simulink model "L1E4pt2_DC_Motor_Speed_Model"  (R2019b)
settings: Solver=VariableStepAuto  StartTime=0.0  StopTime=10.0  RelTol=1e-3
libraries: fl_lib x10, nesl_utility x5
settings Model: Creator=Callum  LastModifiedBy=Callum

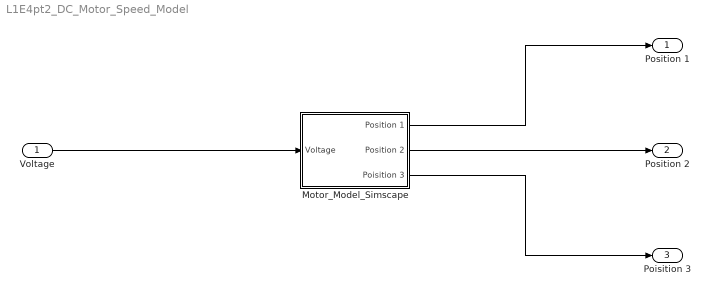
== system L1E4pt2_DC_Motor_Speed_Model ==
  Voltage : Inport
  Motor_Model_Simscape : Subsystem
  Position 1 : Outport
  Position 2 : Outport  Port=2
  Poisition 3 : Outport  Port=3
  wires:
  Voltage/1 -> Motor_Model_Simscape/1(Voltage)
  Motor_Model_Simscape/1(Position 1) -> Position 1/1
  Motor_Model_Simscape/2(Position 2) -> Position 2/1
  Motor_Model_Simscape/3(Poisition 3) -> Poisition 3/1

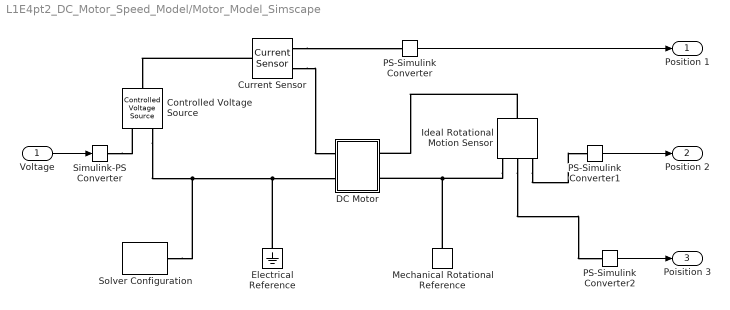
== system L1E4pt2_DC_Motor_Speed_Model/Motor_Model_Simscape ==
  Voltage : Inport
  "Controlled Voltage Source " : fl_lib/Electrical/Electrical Sources/Controlled Voltage Source
  "Current Sensor " : fl_lib/Electrical/Electrical Sensors/Current Sensor
  DC Motor : Subsystem
  "Electrical Reference " : fl_lib/Electrical/Electrical Elements/Electrical Reference
  "Ideal Rotational Motion Sensor " : fl_lib/Mechanical/Mechanical Sensors/Ideal Rotational Motion Sensor  offset=0 rad
  "Mechanical Rotational Reference " : fl_lib/Mechanical/Rotational Elements/Mechanical Rotational Reference
  PS-Simulink Converter : nesl_utility/PS-Simulink Converter  PhysicalDomain=network_engine_domain  SubClassName=ps_output  LeftPortType=input  RightPortType=output  PseudoPeriodic=off  Frequencies=[]  Unit=inherit  AffineConversion=off
  PS-Simulink Converter1 : nesl_utility/PS-Simulink Converter  PhysicalDomain=network_engine_domain  SubClassName=ps_output  LeftPortType=input  RightPortType=output  PseudoPeriodic=off  Frequencies=[]  Unit=inherit  AffineConversion=off
  PS-Simulink Converter2 : nesl_utility/PS-Simulink Converter  PhysicalDomain=network_engine_domain  SubClassName=ps_output  LeftPortType=input  RightPortType=output  PseudoPeriodic=off  Frequencies=[]  Unit=inherit  AffineConversion=off
  "Simulink-PS Converter " : nesl_utility/Simulink-PS Converter  PhysicalDomain=network_engine_domain  SubClassName=ps_input  LeftPortType=input  RightPortType=output  PseudoPeriodic=off  Frequencies=[]  NoiseDistribution=none  NoiseParameters=[]  Unit=1  AffineConversion=off  FilteringAndDerivatives=provide  SimscapeFilterOrder=1  InputFilterTimeConstant=0.001  UdotUserProvided=0
  "Solver Configuration " : nesl_utility/Solver Configuration  PhysicalDomain=network_engine_domain  SubClassName=solver  LeftPortType=input  RightPortType=generic  Tones=[]  Harmonics=[]  SimulateNoise=off  Profile=off  UseLocalSampling=off  EnableSwitchedLinearOptims=on  FrequencyDomain=off  UseCCode=off  RelTol=0.001  AbsTol=1e-06  MinStep=1e-09  ToWorkspace=off  RevertToSquareIcSolve=off  NumHomotopyIterations=100  PhasorMode=off  PhasorModeNumHarmonics=1  DoDC=off  ResidualTolerance=1e-09  UseLocalSolver=off  LocalSolverChoice=NE_BACKWARD_EULER_ADVANCER  LocalSolverSampleTime=0.001  DoFixedCost=off  MaxNonlinIter=3  MaxModeIter=2  LinearAlgebra=auto  EquationFormulation=NE_TIME_EF  DelaysMemoryBudget=1024  AutomaticFiltering=on  FilteringTimeConstant=0.001  PartitionStorageMethod=AS_NEEDED  PartitionMemoryBudget=1024  PartitionMethod=ROBUST
  Position 1 : Outport
  Position 2 : Outport  Port=2
  Poisition 3 : Outport  Port=3
  wires:
  Voltage/1 -> "Simulink-PS Converter "/1
  PS-Simulink Converter/1 -> Position 1/1
  PS-Simulink Converter2/1 -> Poisition 3/1
  PS-Simulink Converter1/1 -> Position 2/1
  connections:
  "Current Sensor "/LConn1 -- "Controlled Voltage Source "/LConn1
  "Current Sensor "/RConn2 -- DC Motor/LConn1
  "Current Sensor "/RConn1 -- PS-Simulink Converter/LConn1
  "Controlled Voltage Source "/RConn2 -- "Solver Configuration "/RConn1 -- "Electrical Reference "/LConn1 -- DC Motor/LConn2
  "Ideal Rotational Motion Sensor "/RConn1 -- "Mechanical Rotational Reference "/LConn1 -- DC Motor/RConn2
  "Ideal Rotational Motion Sensor "/RConn2 -- PS-Simulink Converter2/LConn1
  "Ideal Rotational Motion Sensor "/LConn1 -- DC Motor/RConn1
  "Ideal Rotational Motion Sensor "/RConn3 -- PS-Simulink Converter1/LConn1
  "Simulink-PS Converter "/RConn1 -- "Controlled Voltage Source "/RConn1

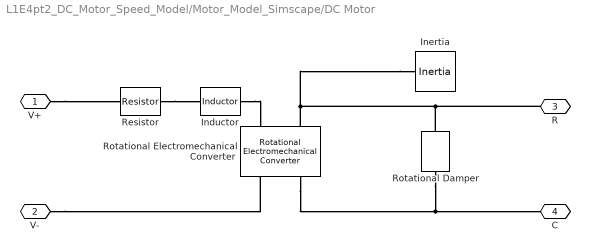
== system L1E4pt2_DC_Motor_Speed_Model/Motor_Model_Simscape/DC Motor ==
  " Inertia" : fl_lib/Mechanical/Rotational Elements/Inertia  inertia=0.01 kg*m^2  w_specify=off  w_priority=High  w=0 rad/s  w_nominal_specify=off  w_nominal_unit=rad/s  w_nominal_value=1  t_specify=off  t_priority=None  t=0 N*m  t_nominal_specify=off  t_nominal_unit=N*m  t_nominal_value=1
  "Inductor " : fl_lib/Electrical/Electrical Elements/Inductor  l=1e-6 H  r=0 Ohm  g=1e-9 1/Ohm  i_specify=off  i_priority=None  i=0 A  i_nominal_specify=off  i_nominal_unit=A  i_nominal_value=1  v_specify=off  v_priority=None  v=0 V  v_nominal_specify=off  v_nominal_unit=V  v_nominal_value=1  i_L_specify=off  i_L_priority=High  i_L=0 A  i_L_nominal_specify=off  i_L_nominal_unit=A  i_L_nominal_value=1
  "Resistor " : fl_lib/Electrical/Electrical Elements/Resistor  R=1 Ohm  i_specify=off  i_priority=None  i=0 A  i_nominal_specify=off  i_nominal_unit=A  i_nominal_value=1  v_specify=off  v_priority=None  v=0 V  v_nominal_specify=off  v_nominal_unit=V  v_nominal_value=1
  "Rotational Electromechanical Converter " : fl_lib/Electrical/Electrical Elements/Rotational Electromechanical Converter  K=0.1 V/(rad/s)  i_specify=off  i_priority=None  i=0 A  i_nominal_specify=off  i_nominal_unit=A  i_nominal_value=1  v_specify=off  v_priority=None  v=0 V  v_nominal_specify=off  v_nominal_unit=V  v_nominal_value=1  t_specify=off  t_priority=None  t=0 N*m  t_nominal_specify=off  t_nominal_unit=N*m  t_nominal_value=1  w_specify=off  w_priority=None  w=0 rad/s  w_nominal_specify=off  w_nominal_unit=rad/s  w_nominal_value=1
      settings: SourceProductName=Simscape
  "Rotational Damper " : fl_lib/Mechanical/Rotational Elements/Rotational Damper  D=0.001 N*m/(rad/s)  w_specify=off  w_priority=None  w=0 rad/s  w_nominal_specify=off  w_nominal_unit=rad/s  w_nominal_value=1  t_specify=off  t_priority=None  t=0 N*m  t_nominal_specify=off  t_nominal_unit=N*m  t_nominal_value=1
  V+ : PMIOPort  Side=Left
  V- : PMIOPort  Port=2  Side=Left
  R : PMIOPort  Port=3  Side=Right
  C : PMIOPort  Port=4  Side=Right
  connections:
  "Inductor "/RConn1 -- "Rotational Electromechanical Converter "/LConn1
  V+/RConn1 -- "Resistor "/LConn1
  " Inertia"/LConn1 -- R/RConn1 -- "Rotational Damper "/RConn1 -- "Rotational Electromechanical Converter "/LConn2
  "Rotational Damper "/LConn1 -- C/RConn1 -- "Rotational Electromechanical Converter "/RConn2
  V-/RConn1 -- "Rotational Electromechanical Converter "/RConn1
  "Resistor "/RConn1 -- "Inductor "/LConn1
